simulink model "problem4"  (R2025b)
settings: Solver=VariableStepAuto  StartTime=0.0  StopTime=9.0  RelTol=1e-3
settings Model: Creator=Maria Islam  LastModifiedBy=Maria Islam

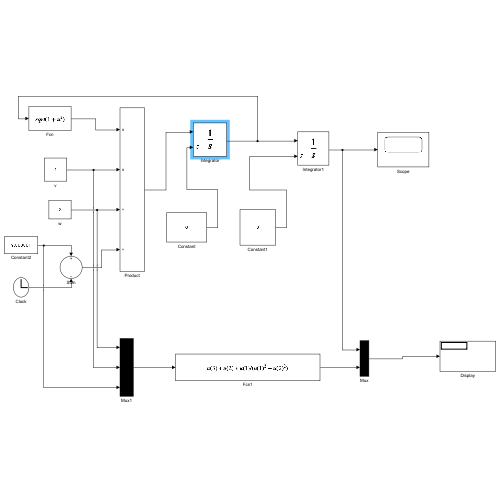
[thumbnail: Simulink's stored preview of the top-level diagram]
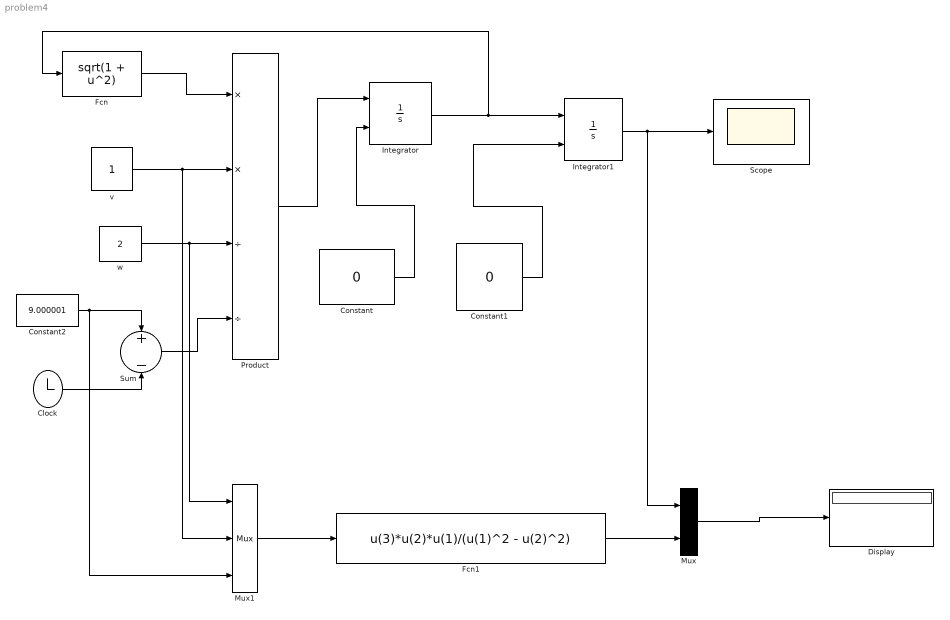
== system problem4 ==
  Clock : Clock
  Constant : Constant  Value=0
  Constant1 : Constant  Value=0
  Constant2 : Constant  Value=9.000001
  Display : Display
  Fcn : Fcn  Expr=sqrt(1 + u^2)
  Fcn1 : Fcn  Expr=u(3)*u(2)*u(1)/(u(1)^2 - u(2)^2)
  Integrator : Integrator  ExternalReset=rising
  Integrator1 : Integrator  ExternalReset=rising
  Mux : Mux  Inputs=2
  Mux1 : Mux  Inputs=3
  Product : Product  Inputs=**//
  Scope : Scope
      settings: ActiveDisplayYMinimum=-0.3937473365849673  ActiveDisplayYMaximum=17.187177902530372
  Sum : Sum  Inputs=+-
  v : Constant
  w : Constant  Value=2
  wires:
  Fcn/1 -> Product/1
  v/1 -> Mux1/2, Product/2
  w/1 -> Mux1/1, Product/3
  Sum/1 -> Product/4
  Constant2/1 -> Mux1/3, Sum/1
  Clock/1 -> Sum/2
  Constant/1 -> Integrator/2
  Constant1/1 -> Integrator1/2
  Product/1 -> Integrator/1
  Integrator/1 -> Fcn/1, Integrator1/1
  Integrator1/1 -> Mux/1, Scope/1
  Mux1/1 -> Fcn1/1
  Fcn1/1 -> Mux/2
  Mux/1 -> Display/1
